simulink model "CSAD_PIDcontroller_ny"  (R2016b)
settings: Solver=ode3  StartTime=0.0  StopTime=tend  FixedStep=0.01  RelTol=1e-3  EnableMultiTasking=on
undefined symbols (not defined in the file): C, Cdn, Cdt, Cmn, d, D, depCur, des_pos, E, emfact, eps_c, epsilon, hd, hd2, Hoerner, I_s, k_cc, K_d_psi, K_d_x, K_d_y, K_i_psi, K_i_x, K_i_y, K_omega, K_p_psi, K_p_x, K_p_y, Kp, Kq, Kqr, Kt, Ktr, L, Max_Acceleration, Max_rotation, Max_thrust, moorLineProp, n_c, n_max, p_cc, P_max, Q_f0, Q_max, r0, r_cc, r_dot0, rBottomEnd, Rho, rhoCab, rhoWat, stiffSeafloor, T_psi, T_x, T_y, Thruster, Thruster_control, Thruster_lock, velCur, vessel, vesselABC ... (+7)
libraries: marine_gnc x9, dspmtrx3 x6, simulink x6, simulink_extras x3, marine_hydro x3
(part 1 of 5)
settings Model: Creator=JonBjoernoe  LastModifiedBy=silje
settings SolverCC: AlgebraicLoopSolver=LineSearch
settings OptimizationCC: LifeSpan=inf
settings DebuggingCC: SFUnexpectedBacktrackingDiag=warning  SFNoUnconditionalDefaultTransitionDiag=warning  SFExecutionAtInitializationDiag=none
settings ModelReferenceCC: ModelReferenceMinAlgLoopOccurrences=on
settings GRTTargetCC: TargetLangStandard=C89/C90 (ANSI)  GeneratePreprocessorConditionals=Disable all
settings ConfigComp: CovMetricSettings=dw  CovHtmlReporting=on  CovSaveCumulativeToWorkspaceVar=on  CovSaveSingleToWorkspaceVar=on  CovExternalEMLEnable=off

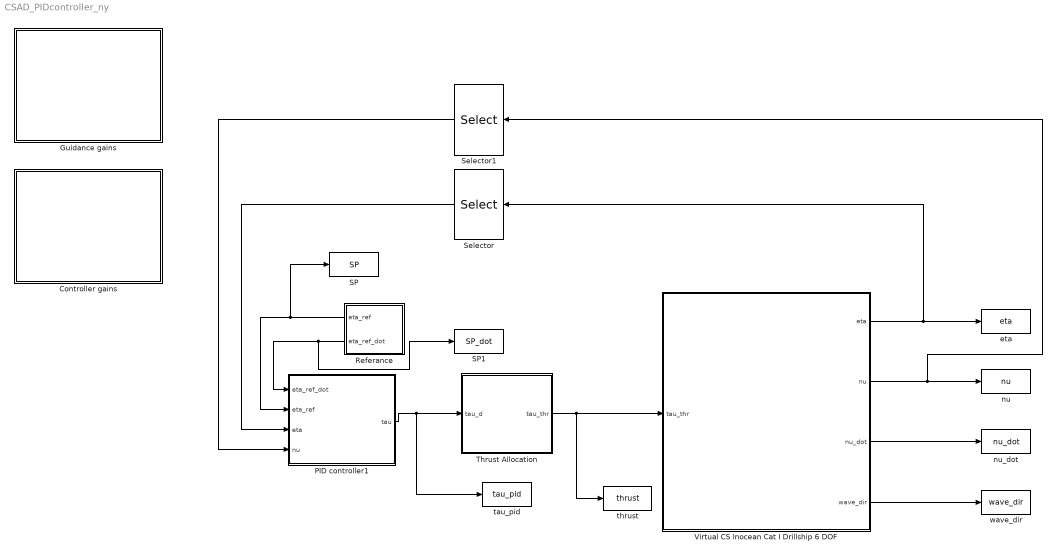
== system CSAD_PIDcontroller_ny ==
  Controller gains : Subsystem
  Guidance gains : Subsystem
  PID controller1 : Subsystem
  Referance : Subsystem
  SP : ToWorkspace  VariableName=SP  SaveFormat=Timeseries  SampleTime=-1
  SP1 : ToWorkspace  VariableName=SP_dot  SaveFormat=Timeseries  SampleTime=-1
  Selector : Selector  InputPortWidth=6  IndexOptions=Index vector (dialog)  Indices=[1 2 6]  OutputSizes=1
  Selector1 : Selector  InputPortWidth=6  IndexOptions=Index vector (dialog)  Indices=[1 2 6]  OutputSizes=1
  "Thrust Allocation  " : Subsystem
  Virtual CS Inocean Cat I Drillship 6 DOF : Subsystem  mask(CSAD with Turret-based thruster-assisted position mooring){eta_0=[0 0 0 0 0 0], nu_0=[0 0 0 0 0 0], wave_1_on_off=off, wave_2_on_off=on, Hs=1.5/90, beta_w=3.4907, omega_0=0.768*sqrt(90), current_on_off=on, nu_c=0.2/sqrt(90), beta_c=200, anchor_0=moorLineProp.bottomEnds, mooringLinesMeasurement_on_off=off, mooringLines_on_off=off}
      mask prompts: eta_0 "Initial eta"; nu_0 "Initial nu"; wave_1_on_off "Wave force (1st Order)"; wave_2_on_off "Wave drift force (2nd Order)"; Hs "Significant wave height [m] (Hs)"; beta_w "Mean wave direction [rad] (beta_w)"; omega_0 "Peak frequency [rad/s] (omega_0)"; current_on_off "Current"; nu_c "Current velocity [m/s] (nu_c)"; beta_c "Current direction [deg] (beta_c)"; anchor_0 "The anchor position matrix"; mooringLinesMeasurement_on_off "Mooring Lines' Measurement"; mooringLines_on_off "Mooring Lines"
      mask help:
      | This block implements the CS Inocean Cat I Drillship with 4 mooring lines. This is a simplified model. All the mooring lines are assumed to connect with the turret at the center of the turret (COT). The COT locates at the center of the ship.  Therefore, there are no moments from mooring lines.
      |
      | where
      | input 1:     <tau_thr> Thruster forces.
      | output 1:   <Wave direction> The direction of the waves.
      | output 2:   <eta> The position of the CSAD.
      | output 3:   <nu> The velocity of the CSAD.
      | output 4:   <T_moor> The tension vector in every mooring line.
      |
      | Copyright (C) 2016, NTNU, Trondheim, Norway
      | Author: Jon Bjørnø (CSAD) and Zhengru Ren (mooring)
  eta : ToWorkspace  VariableName=eta  SaveFormat=Timeseries  SampleTime=-1
  nu : ToWorkspace  VariableName=nu  SaveFormat=Timeseries  SampleTime=-1
  nu_dot : ToWorkspace  VariableName=nu_dot  SaveFormat=Timeseries  SampleTime=-1
  tau_pid : ToWorkspace  VariableName=tau_pid  SaveFormat=Timeseries  SampleTime=-1
  thrust : ToWorkspace  VariableName=thrust  SaveFormat=Timeseries  SampleTime=-1
  wave_dir : ToWorkspace  VariableName=wave_dir  SaveFormat=Timeseries  SampleTime=-1
  wires:
  Virtual CS Inocean Cat I Drillship 6 DOF/1(eta) -> Selector/1, eta/1
  Virtual CS Inocean Cat I Drillship 6 DOF/2(nu) -> nu/1, Selector1/1
  Virtual CS Inocean Cat I Drillship 6 DOF/3(nu_dot) -> nu_dot/1
  Virtual CS Inocean Cat I Drillship 6 DOF/4(wave_dir) -> wave_dir/1
  "Thrust Allocation  "/1(tau_thr) -> thrust/1, Virtual CS Inocean Cat I Drillship 6 DOF/1(tau_thr)
  PID controller1/1(tau) -> tau_pid/1, "Thrust Allocation  "/1(tau_d)
  Selector/1 -> PID controller1/3(eta)
  Selector1/1 -> PID controller1/4(nu)
  Referance/1(eta_ref) -> SP/1, PID controller1/2(eta_ref)
  Referance/2(eta_ref_dot) -> SP1/1, PID controller1/1(eta_ref_dot)

== system CSAD_PIDcontroller_ny/Controller gains ==
  Constant : Constant  Value=K_p_x
  Constant1 : Constant  Value=K_p_y
  Constant2 : Constant  Value=K_p_psi
  Constant3 : Constant  Value=K_i_x
  Constant4 : Constant  Value=K_i_y
  Constant5 : Constant  Value=K_i_psi
  Constant6 : Constant  Value=K_d_x
  Constant7 : Constant  Value=K_d_y
  Constant8 : Constant  Value=K_d_psi
  Create Diagonal Matrix : dspmtrx3/Create Diagonal Matrix
  Create Diagonal Matrix1 : dspmtrx3/Create Diagonal Matrix
  Create Diagonal Matrix2 : dspmtrx3/Create Diagonal Matrix
  Mux : Mux  Inputs=3
  Mux1 : Mux  Inputs=3
  Mux2 : Mux  Inputs=3
  tag scope: K_d=global, K_i=global, K_p=global
  wires:
  Mux/1 -> Create Diagonal Matrix/1
  Constant/1 -> Mux/1
  Constant1/1 -> Mux/2
  Constant2/1 -> Mux/3
  Mux1/1 -> Create Diagonal Matrix1/1
  Create Diagonal Matrix/1 -> [K_p]
  Create Diagonal Matrix1/1 -> [K_i]
  Mux2/1 -> Create Diagonal Matrix2/1
  Create Diagonal Matrix2/1 -> [K_d]
  Constant3/1 -> Mux1/1
  Constant4/1 -> Mux1/2
  Constant5/1 -> Mux1/3
  Constant6/1 -> Mux2/1
  Constant7/1 -> Mux2/2
  Constant8/1 -> Mux2/3

== system CSAD_PIDcontroller_ny/Guidance gains ==
  Constant : Constant  Value=w_x
  Constant1 : Constant  Value=w_y
  Constant2 : Constant  Value=w_psi
  Constant3 : Constant  Value=zeta_x
  Constant4 : Constant  Value=zeta_y
  Constant5 : Constant  Value=zeta_psi
  Constant6 : Constant  Value=1/T_x
  Constant7 : Constant  Value=1/T_y
  Constant8 : Constant  Value=1/T_psi
  Create Diagonal Matrix : dspmtrx3/Create Diagonal Matrix
  Create Diagonal Matrix1 : dspmtrx3/Create Diagonal Matrix
  Create Diagonal Matrix2 : dspmtrx3/Create Diagonal Matrix
  Mux : Mux  Inputs=3
  Mux1 : Mux  Inputs=3
  Mux2 : Mux  Inputs=3
  tag scope: Af=global, omega=global, zeta=global
  wires:
  Mux/1 -> Create Diagonal Matrix/1
  Constant/1 -> Mux/1
  Constant1/1 -> Mux/2
  Constant2/1 -> Mux/3
  Mux1/1 -> Create Diagonal Matrix1/1
  Constant3/1 -> Mux1/1
  Constant4/1 -> Mux1/2
  Constant5/1 -> Mux1/3
  Create Diagonal Matrix/1 -> [omega]
  Create Diagonal Matrix1/1 -> [zeta]
  Mux2/1 -> Create Diagonal Matrix2/1
  Constant6/1 -> Mux2/1
  Constant7/1 -> Mux2/2
  Constant8/1 -> Mux2/3
  Create Diagonal Matrix2/1 -> [Af]

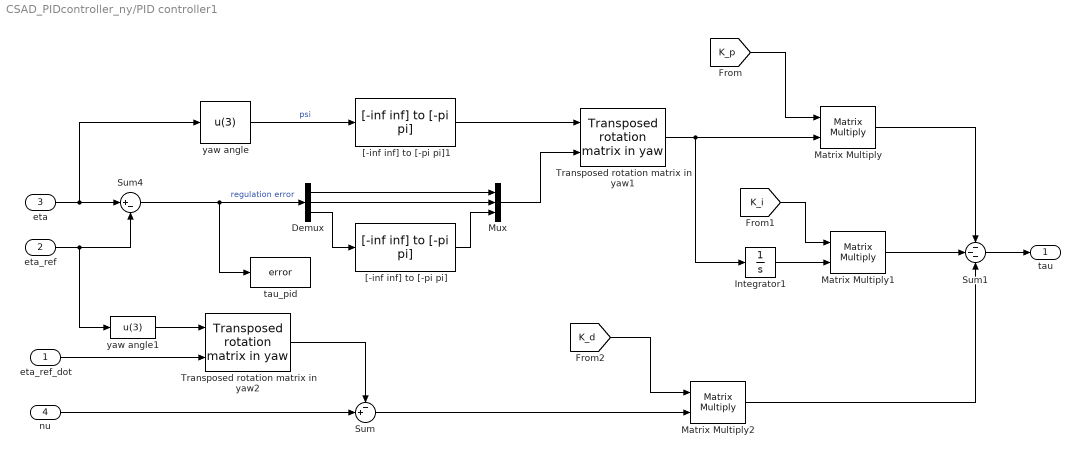
== system CSAD_PIDcontroller_ny/PID controller1 ==
  eta_ref_dot : Inport
  eta_ref : Inport  Port=2
  eta : Inport  Port=3
  nu : Inport  Port=4
  Demux : Demux  Outputs=3
  Integrator1 : Integrator
  Matrix Multiply : Product  Multiplication=Matrix(*)
  Matrix Multiply1 : Product  Multiplication=Matrix(*)
  Matrix Multiply2 : Product  Multiplication=Matrix(*)
  Mux : Mux  Inputs=3
  Sum : Sum  Inputs=-+|
  Sum1 : Sum  Inputs=---  SaturateOnIntegerOverflow=on  InputSameDT=on  OutDataTypeStr=Inherit: Same as first input
  Sum4 : Sum  Inputs=|+-  SaturateOnIntegerOverflow=on  InputSameDT=on  OutDataTypeStr=Inherit: Same as first input
  Transposed rotation matrix in yaw1 : marine_gnc/Models/ Kinematics/Transposed rotation  matrix in yaw
  Transposed rotation matrix in yaw2 : marine_gnc/Models/ Kinematics/Transposed rotation  matrix in yaw
  "[-inf inf] to [-pi pi]" : marine_gnc/Utilities/Math Operations/[-inf inf] to [-pi pi]
  "[-inf inf] to [-pi pi]1" : marine_gnc/Utilities/Math Operations/[-inf inf] to [-pi pi]
  tau_pid : ToWorkspace  VariableName=error  SaveFormat=Timeseries  SampleTime=-1
  yaw angle : Fcn  Expr=u(3)
  yaw angle1 : Fcn  Expr=u(3)
  tau : Outport  InitialOutput=0
  wires:
  Demux/2 -> Mux/2
  Demux/1 -> Mux/1
  Mux/1 -> Transposed rotation matrix in yaw1/2
  Sum4/1 -> tau_pid/1, Demux/1  "regulation error"
  "[-inf inf] to [-pi pi]"/1 -> Mux/3
  yaw angle/1 -> "[-inf inf] to [-pi pi]1"/1  "psi"
  "[-inf inf] to [-pi pi]1"/1 -> Transposed rotation matrix in yaw1/1
  Demux/3 -> "[-inf inf] to [-pi pi]"/1
  Transposed rotation matrix in yaw1/1 -> Matrix Multiply/2, Integrator1/1
  Sum1/1 -> tau/1
  eta_ref/1 -> yaw angle1/1, Sum4/2
  eta/1 -> yaw angle/1, Sum4/1
  [K_p] -> Matrix Multiply/1
  Matrix Multiply/1 -> Sum1/1
  Integrator1/1 -> Matrix Multiply1/2
  Matrix Multiply1/1 -> Sum1/2
  [K_i] -> Matrix Multiply1/1
  [K_d] -> Matrix Multiply2/1
  Matrix Multiply2/1 -> Sum1/3
  eta_ref_dot/1 -> Transposed rotation matrix in yaw2/2
  yaw angle1/1 -> Transposed rotation matrix in yaw2/1
  nu/1 -> Sum/2
  Sum/1 -> Matrix Multiply2/2
  Transposed rotation matrix in yaw2/1 -> Sum/1

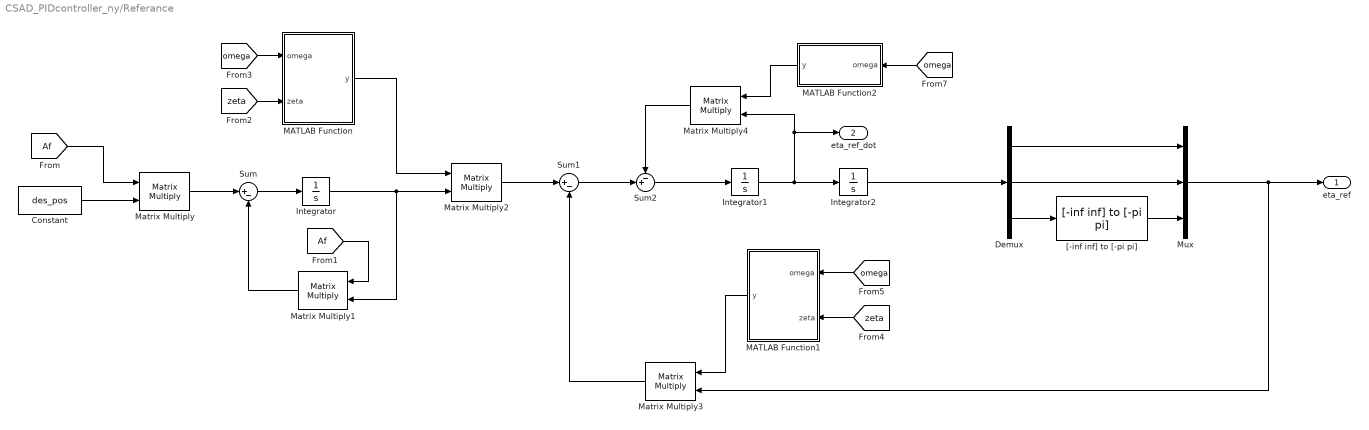
== system CSAD_PIDcontroller_ny/Referance ==
  Constant : Constant  Value=des_pos
  Demux : Demux  Outputs=3
  Integrator : Integrator
  Integrator1 : Integrator
  Integrator2 : Integrator
  MATLAB Function : MATLAB Function  TreatAsAtomicUnit=on
  MATLAB Function1 : MATLAB Function  TreatAsAtomicUnit=on
  MATLAB Function2 : MATLAB Function  TreatAsAtomicUnit=on
  Matrix Multiply{,1..4} (5 alike) : Product  Multiplication=Matrix(*)
  Mux : Mux  Inputs=3
  Sum : Sum  Inputs=|+-
  Sum1 : Sum  Inputs=|+-
  Sum2 : Sum  Inputs=-+|
  "[-inf inf] to [-pi pi]" : marine_gnc/Utilities/Math Operations/[-inf inf] to [-pi pi]
  eta_ref : Outport
  eta_ref_dot : Outport  Port=2
  wires:
  Constant/1 -> Matrix Multiply/2
  [Af] -> Matrix Multiply/1
  Matrix Multiply/1 -> Sum/1
  Sum/1 -> Integrator/1
  Matrix Multiply1/1 -> Sum/2
  [Af] -> Matrix Multiply1/1
  Integrator/1 -> Matrix Multiply2/2, Matrix Multiply1/2
  [zeta] -> MATLAB Function/2(zeta)
  [omega] -> MATLAB Function/1(omega)
  MATLAB Function/1(y) -> Matrix Multiply2/1
  Matrix Multiply2/1 -> Sum1/1
  Sum1/1 -> Sum2/2
  Sum2/1 -> Integrator1/1
  Integrator1/1 -> eta_ref_dot/1, Matrix Multiply4/2, Integrator2/1
  [zeta] -> MATLAB Function1/2(zeta)
  [omega] -> MATLAB Function1/1(omega)
  MATLAB Function1/1(y) -> Matrix Multiply3/1
  Matrix Multiply3/1 -> Sum1/2
  [omega] -> MATLAB Function2/1(omega)
  MATLAB Function2/1(y) -> Matrix Multiply4/1
  Matrix Multiply4/1 -> Sum2/1
  Demux/3 -> "[-inf inf] to [-pi pi]"/1
  "[-inf inf] to [-pi pi]"/1 -> Mux/3
  Demux/2 -> Mux/2
  Demux/1 -> Mux/1
  Integrator2/1 -> Demux/1
  Mux/1 -> Matrix Multiply3/2, eta_ref/1

== system CSAD_PIDcontroller_ny/Thrust Allocation   ==
  tau_d : Inport
  "Parameters From initfile distributed " : Subsystem
  T(F,alpha) : Subsystem
  Thrust allocation1 : Subsystem
  "Thruster control " : Subsystem
  tau_thr : Outport
  wires:
  T(F,alpha)/1(Commanded tau) -> tau_thr/1
  tau_d/1 -> Thrust allocation1/1(tau)
  "Thruster control "/2(Commanded angle) -> T(F,alpha)/2(Commanded angle), Thrust allocation1/2(Angles)
  Thrust allocation1/1(Td & angle) -> "Thruster control "/1("Desired thrust and angle ")
  "Thruster control "/1("Commanded thrust ") -> T(F,alpha)/1(Commanded thrust)

== system CSAD_PIDcontroller_ny/Virtual CS Inocean Cat I Drillship 6 DOF ==
  tau_thr : Inport
  3 to 6 DOF : marine_gnc/Models/ Kinetics /Support/3 to 6 DOF  SystemSampleTime=-1
  6 DOF DP model (zero speed model with fluid memory) : Subsystem  mask(6 DOF zero speed model){ABC=vesselABC, rho=1025, Axc=0.9*vessel.main.T*vessel.main.B, Ayc=0.9*vessel.main.T*vessel.main.Lpp, CX=1, CY_2D=Hoerner(vessel.main.B,vessel.main.T), Bv=vessel.Bv(:,:,1)}
      mask prompts: ABC "Structure containing model parameters and the fluid memory effects"; rho "Density of water (kg/m3)"; Axc "Frontal projected current area Axc (m2)"; Ayc "Laterall projected current area Ayc (m2)"; CX "Current (drag) coefficient in surge CX"; CY_2D "2D drag coefficient in sway CY_2D"; Bv "Linear viscous damping matrix"
      mask help: System block containing the zero speed 6 DOF equations of motion including fluid memory effetcs.
  Current : Subsystem
  Current direction (deg) : Constant  Value=beta_c
  Current speed (m/s) : Constant  Value=nu_c
  FEM mooring : Subsystem  mask(Mooring Force Model){r_0=moorLineProp.bottomEnds}
      mask prompts: r_0 "The anchor position matrix"
      mask help:
      | This block implements the mooring forces with catenary equations. There are 8 mooring lines in this mooring system. This is a simplified model. All the mooring lines are assumed to connect with the turret at the center of the turret (COT). The COT locates at the center of the ship.  Therefore, there are no moments from mooring lines.
      |
      | where
      | input 1:    <eta> The position of the turrent terminal point.
      | output 1:   <tau_moor> The total mooring forces in 6DOF. The moments in roll, pitch, and yaw are zeros.
      | output 2:   <T_moor> The tension vector in every mooring lines.
      |
      | Copyright (C) 2015, NTNU, Trondheim, Norway
      | Author: Zhengru Ren
      | Edited: Jon Bjørnø 2016
      mask DialogControl Container2 Prompt: Parameters
  Waves : Subsystem
  current : ToWorkspace  VariableName=current  SaveFormat=Timeseries  SampleTime=-1
  "currentForce on/off " : Gain  Gain=current_on_off
  mooringLines on/off : Gain  Gain=mooringLines_on_off
  wave : ToWorkspace  VariableName=wave  SaveFormat=Timeseries  SampleTime=-1
  eta : Outport
  nu : Outport  Port=2
  nu_dot : Outport  Port=3
  wave_dir : Outport  Port=4
  wires:
  6 DOF DP model (zero speed model with fluid memory)/2(nu) -> nu/1
  tau_thr/1 -> 3 to 6 DOF/1
  3 to 6 DOF/1 -> 6 DOF DP model (zero speed model with fluid memory)/2(tau_thr)
  FEM mooring/1(tau_moor) -> mooringLines on/off/1
  "currentForce on/off "/1 -> current/1, 6 DOF DP model (zero speed model with fluid memory)/3(nu_c)
  Current/1(nu_c) -> "currentForce on/off "/1
  Current speed (m/s)/1 -> Current/2(V_c (m/s))
  Current direction (deg)/1 -> Current/1(beta_c (deg))
  6 DOF DP model (zero speed model with fluid memory)/3(nu_dot) -> nu_dot/1
  6 DOF DP model (zero speed model with fluid memory)/1(eta) -> Waves/1(eta), FEM mooring/1(eta), eta/1
  Waves/1(wave_dir) -> wave_dir/1
  Waves/2(tau_wave) -> wave/1, 6 DOF DP model (zero speed model with fluid memory)/1(tau_wave)
  mooringLines on/off/1 -> 6 DOF DP model (zero speed model with fluid memory)/4(tau_mooring)

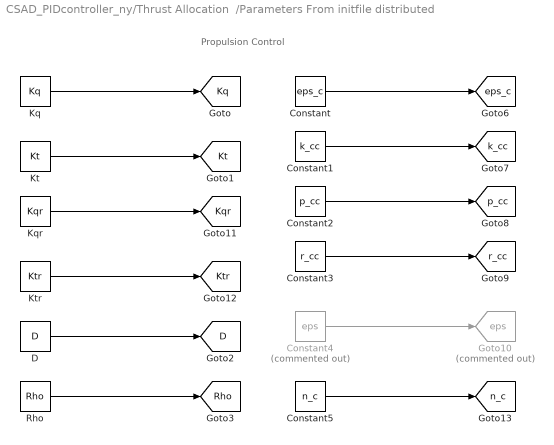
== system CSAD_PIDcontroller_ny/Thrust Allocation  /Parameters From initfile distributed  ==
  note: Propulsion Control
  Constant : Constant  Value=eps_c
  Constant1 : Constant  Value=k_cc
  Constant2 : Constant  Value=p_cc
  Constant3 : Constant  Value=r_cc
  Constant4 : Constant  Commented=on  Value=eps
  Constant5 : Constant  Value=n_c
  D : Constant  Value=D
  Goto10 : Goto  Commented=on  GotoTag=eps  TagVisibility=global
  Kq : Constant  Value=Kq
  Kqr : Constant  Value=Kqr
  Kt : Constant  Value=Kt
  Ktr : Constant  Value=Ktr
  Rho : Constant  Value=Rho
  tag scope: D=global, Kq=global, Kqr=global, Kt=global, Ktr=global, Rho=global, eps_c=global, k_cc=global, n_c=global, p_cc=global, r_cc=global
  wires:
  Kq/1 -> [Kq]
  Kt/1 -> [Kt]
  D/1 -> [D]
  Rho/1 -> [Rho]
  Constant/1 -> [eps_c]
  Constant1/1 -> [k_cc]
  Constant2/1 -> [p_cc]
  Constant3/1 -> [r_cc]
  Constant4/1 -> Goto10/1
  Kqr/1 -> [Kqr]
  Ktr/1 -> [Ktr]
  Constant5/1 -> [n_c]

== system CSAD_PIDcontroller_ny/Thrust Allocation  /T(F,alpha) ==
  Commanded thrust : Inport
  Commanded angle : Inport  Port=2
  MATLAB Function : MATLAB Function  TreatAsAtomicUnit=on
  Radians to Degrees : simulink_extras/Transformations/Radians to Degrees
  X-position Thruster : Constant  Value=[Thruster.T1(1) Thruster.T2(1) Thruster.T3(1) Thruster.T4(1) Thruster.T5(1) Thruster.T6(1)]
  Y-position Thruster : Constant  Value=[Thruster.T1(2) Thruster.T2(2) Thruster.T3(2) Thruster.T4(2) Thruster.T5(2) Thruster.T6(2)]
  Commanded tau : Outport
  wires:
  Commanded angle/1 -> Radians to Degrees/1
  X-position Thruster/1 -> MATLAB Function/3(PosX)
  Y-position Thruster/1 -> MATLAB Function/4(PosY)
  MATLAB Function/1(actual_tau) -> Commanded tau/1
  Commanded thrust/1 -> MATLAB Function/1(thrust_actual)
  Radians to Degrees/1 -> MATLAB Function/2(alpha_actual)

== system CSAD_PIDcontroller_ny/Thrust Allocation  /Thrust allocation1 ==
  tau : Inport
  Angles : Inport  Port=2
  "  Thrust calculated" : Selector  InputPortWidth=12  IndexOptions=Index vector (dialog)  Indices=[7 8 9 10 11 12]  OutputSizes=1
  " Angle calculated" : Selector  InputPortWidth=12  IndexOptions=Index vector (dialog)  Indices=[1 2 3 4 5 6]  OutputSizes=1
  Choosing Fixed / Azimuth angle : Switch  Threshold=1
  Constant to avoid singularities : Constant  Value=eps
  For Each Subsystem : Subsystem  TreatAsAtomicUnit=on
  Mux : Mux  Inputs=3
  Mux2 : Mux  Inputs=2
  Radians to Degrees : simulink_extras/Transformations/Radians to Degrees
  Switch Azimuth/Fixed angles : Constant  Value=Thruster_lock
  Thrust and angle specified : Selector  InputPortWidth=12  IndexOptions=Index vector (dialog)  Indices=[7 1 8 2 9 3 10 4 11 5 12 6]  OutputSizes=1
  ThrustAllocation_Pseudoinverse : S-Function  FunctionName=thrustallocationPseudo  Parameters=Thruster,C  SFunctionDeploymentMode=off  EnableBusSupport=off
      settings: AttributesFormatString=%<Commented>
  constant angle : Constant  Value=[Thruster.T1(3) Thruster.T2(3) Thruster.T3(3) Thruster.T4(3) Thruster.T5(3) Thruster.T6(3)]
  Td & angle : Outport
  wires:
  Switch Azimuth/Fixed angles/1 -> Choosing Fixed / Azimuth angle/2
  Constant to avoid singularities/1 -> Mux/3
  " Angle calculated"/1 -> Choosing Fixed / Azimuth angle/1
  Thrust and angle specified/1 -> Td & angle/1
  Mux2/1 -> Thrust and angle specified/1
  tau/1 -> Mux/1
  Choosing Fixed / Azimuth angle/1 -> For Each Subsystem/1(Desired Angle)
  Angles/1 -> Radians to Degrees/1
  For Each Subsystem/1("angle ") -> Mux2/1
  constant angle/1 -> For Each Subsystem/2("initial angle "), Choosing Fixed / Azimuth angle/3
  Radians to Degrees/1 -> Mux/2
  ThrustAllocation_Pseudoinverse/1 -> " Angle calculated"/1, "  Thrust calculated"/1
  Mux/1 -> ThrustAllocation_Pseudoinverse/1
  "  Thrust calculated"/1 -> Mux2/2

== system CSAD_PIDcontroller_ny/Thrust Allocation  /Thruster control  ==
  "Desired thrust and angle " : Inport
  Demux : Demux  Outputs=12
  Mux : Mux  Inputs=12
  Selecting Actual thrust : Selector  InputPortWidth=12  IndexOptions=Index vector (dialog)  Indices=[1 3 5 7 9 11]  OutputSizes=1
  Selecting actual angle : Selector  InputPortWidth=12  IndexOptions=Index vector (dialog)  Indices=[2 4 6 8 10 12]  OutputSizes=1
  Subsystem : Subsystem
  Subsystem1 : Subsystem  Commented=through
  Thruster 1 : Subsystem
      settings: AttributesFormatString=%<MinAlgLoopOccurrences>
  Thruster 2 : Subsystem
      settings: AttributesFormatString=%<MinAlgLoopOccurrences>
  Thruster 3 : Subsystem
      settings: AttributesFormatString=%<MinAlgLoopOccurrences>
  Thruster 4 : Subsystem
      settings: AttributesFormatString=%<MinAlgLoopOccurrences>
  Thruster 5 : Subsystem
      settings: AttributesFormatString=%<MinAlgLoopOccurrences>
  Thruster 6 : Subsystem
      settings: AttributesFormatString=%<MinAlgLoopOccurrences>
  "Commanded thrust " : Outport
  Commanded angle : Outport  Port=2
  wires:
  "Desired thrust and angle "/1 -> Demux/1
  Demux/3 -> Thruster 2/1(Desired thrust 1)
  Demux/4 -> Thruster 2/2(Desired Angle)
  Demux/5 -> Thruster 3/1(Desired thrust 1)
  Demux/6 -> Thruster 3/2(Desired Angle)
  Demux/7 -> Thruster 4/1(Desired thrust 1)
  Demux/8 -> Thruster 4/2(Desired Angle)
  Demux/9 -> Thruster 5/1(Desired thrust 1)
  Demux/10 -> Thruster 5/2(Desired Angle)
  Demux/11 -> Thruster 6/1(Desired thrust 1)
  Demux/12 -> Thruster 6/2(Desired Angle)
  Thruster 1/1(Commanded thrust 1) -> Mux/1
  Thruster 2/1(Commanded thrust 1) -> Mux/3
  Thruster 2/2(Commanded angle) -> Mux/4
  Thruster 3/1("Commanded thrust ") -> Mux/5
  Thruster 3/2(Commanded angle) -> Mux/6
  Thruster 4/1("Commanded thrust ") -> Mux/7
  Thruster 4/2(Commanded angle) -> Mux/8
  Thruster 5/1(Commanded thrust 1) -> Mux/9
  Thruster 5/2(Commanded angle) -> Mux/10
  Thruster 6/1(Commanded thrust 1) -> Mux/11
  Thruster 6/2(Commanded angle) -> Mux/12
  Selecting actual angle/1 -> Subsystem1/1(Calculated angles)
  Mux/1 -> Selecting Actual thrust/1, Selecting actual angle/1
  Demux/2 -> Thruster 1/2(Desired Angle)
  Thruster 1/2(Commanded angle) -> Mux/2
  Subsystem1/1(Commanded angles) -> Commanded angle/1
  Subsystem/1(Thrust from model) -> "Commanded thrust "/1
  Selecting Actual thrust/1 -> Subsystem/1(Calculated thrust)
  Demux/1 -> Thruster 1/1(Desired thrust 1)

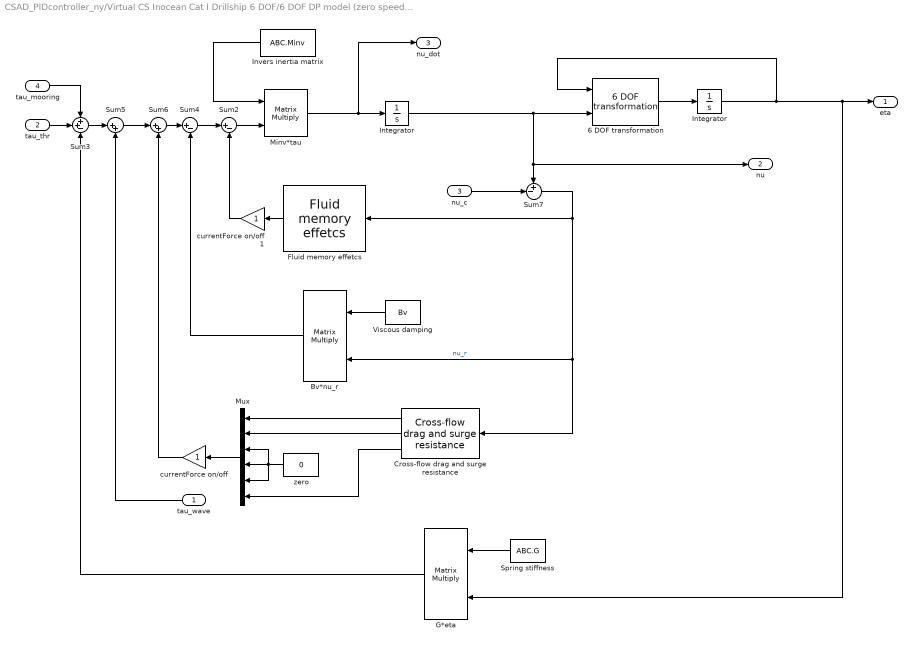
== system CSAD_PIDcontroller_ny/Virtual CS Inocean Cat I Drillship 6 DOF/6 DOF DP model (zero speed model with fluid memory) ==
  tau_wave : Inport
  tau_thr : Inport  Port=2
  nu_c : Inport  Port=3
  tau_mooring : Inport  Port=4
  6 DOF transformation : marine_gnc/Models/ Kinematics/6 DOF transformation
  Bv*nu_r : Product  Multiplication=Matrix(*)  SaturateOnIntegerOverflow=on  OutDataTypeStr=Inherit: Same as first input
  Cross-flow drag and surge resistance : marine_hydro/Hydro Library/Cross-flow drag and surge resistance  N=20  Lpp=vessel.main.Lpp  CD=CY_2D  Cx=CX  Ax=Axc  Ay=Ayc  rho_w=rho
  Fluid memory effetcs : marine_hydro/Hydro Library/6 DOF DP model  (zero speed model with fluid memory)/Fluid memory effetcs
  G*eta : Product  Multiplication=Matrix(*)  SaturateOnIntegerOverflow=on  OutDataTypeStr=Inherit: Same as first input
  Integrator : Integrator  InitialCondition=eta_0
  "Integrator " : Integrator  InitialCondition=nu_0
  Invers inertia matrix : Constant  Value=ABC.Minv
  Minv*tau : Product  Inputs=**  Multiplication=Matrix(*)  SaturateOnIntegerOverflow=on  OutDataTypeStr=Inherit: Same as first input
  Mux : Mux  Inputs=6
  Spring stiffness : Constant  Value=ABC.G
  Sum2 : Sum  Inputs=|+-  SaturateOnIntegerOverflow=on
  Sum3 : Sum  Inputs=++-  SaturateOnIntegerOverflow=on
  Sum4 : Sum  Inputs=|+-  SaturateOnIntegerOverflow=on
  Sum5 : Sum  Inputs=|++  SaturateOnIntegerOverflow=on
  Sum6 : Sum  Inputs=|++  SaturateOnIntegerOverflow=on
  Sum7 : Sum  Inputs=+-|  SaturateOnIntegerOverflow=on
  Viscous damping : Constant  Value=Bv
  "currentForce on/off " : Gain
  currentForce on/off 1 : Gain
  zero : Constant  Value=0
  eta : Outport
  nu : Outport  Port=2
  nu_dot : Outport  Port=3
  wires:
  6 DOF transformation/1 -> Integrator/1
  Cross-flow drag and surge resistance/1 -> Mux/1
  tau_wave/1 -> Sum5/2
  Sum5/1 -> Sum6/1
  Integrator/1 -> 6 DOF transformation/1, eta/1, G*eta/2
  Spring stiffness/1 -> G*eta/1
  Sum6/1 -> Sum4/1
  "Integrator "/1 -> 6 DOF transformation/2, nu/1, Sum7/1
  Sum7/1 -> Fluid memory effetcs/1, Cross-flow drag and surge resistance/1, Bv*nu_r/2  "nu_r"
  Mux/1 -> "currentForce on/off "/1
  Viscous damping/1 -> Bv*nu_r/1
  Sum4/1 -> Sum2/1
  Cross-flow drag and surge resistance/3 -> Mux/6
  zero/1 -> Mux/4, Mux/3, Mux/5
  Sum2/1 -> Minv*tau/2
  Sum3/1 -> Sum5/1
  Fluid memory effetcs/1 -> currentForce on/off 1/1
  Invers inertia matrix/1 -> Minv*tau/1
  nu_c/1 -> Sum7/2
  Bv*nu_r/1 -> Sum4/2
  Cross-flow drag and surge resistance/2 -> Mux/2
  Minv*tau/1 -> nu_dot/1, "Integrator "/1
  tau_thr/1 -> Sum3/2
  tau_mooring/1 -> Sum3/1
  "currentForce on/off "/1 -> Sum6/2
  currentForce on/off 1/1 -> Sum2/2
  G*eta/1 -> Sum3/3

== system CSAD_PIDcontroller_ny/Virtual CS Inocean Cat I Drillship 6 DOF/Current ==
  beta_c (deg) : Inport
  V_c (m/s) : Inport  Port=2
  Gain : Gain  Gain=pi/180
  Mux : Mux  Inputs=6
  Product : Product  RndMeth=Zero
  Product1 : Product  RndMeth=Zero
  cos : Trigonometry  Operator=cos
  deg to 180/180 : marine_gnc/Utilities/Math Operations/deg to 180//180
  sin : Trigonometry
  zero : Constant  Value=0
  nu_c : Outport
  wires:
  sin/1 -> Product1/1
  cos/1 -> Product/1
  Product1/1 -> Mux/2
  zero/1 -> Mux/6, Mux/5, Mux/4, Mux/3
  V_c (m/s)/1 -> Product/2, Product1/2
  Gain/1 -> cos/1, sin/1
  Product/1 -> Mux/1
  Mux/1 -> nu_c/1
  beta_c (deg)/1 -> deg to 180/180/1
  deg to 180/180/1 -> Gain/1

== system CSAD_PIDcontroller_ny/Virtual CS Inocean Cat I Drillship 6 DOF/FEM mooring ==
  eta : Inport
  3 DOF transformation : MATLAB Function  TreatAsAtomicUnit=on
  Gain{,1..3} (4 alike) : Gain  Gain=0
  Mooring Line 1 : Subsystem
  Mooring Line 2 : Subsystem
  Mooring Line 3 : Subsystem
  Mooring Line 4 : Subsystem
  Mooring Line 5 : Subsystem
  Mooring Line 6 : Subsystem
  Mooring Line 7 : Subsystem
  Mooring Line 8 : Subsystem
  Selector : Selector  InputPortWidth=6  IndexOptions=Index vector (dialog)  Indices=[1 2 3]  OutputSizes=1
  Sum1 : Sum  Inputs=++++++++  SaturateOnIntegerOverflow=on  InputSameDT=on  OutDataTypeStr=Inherit: Same as first input
  eta1 : InportShadow
  mooring : ToWorkspace  VariableName=mooring  SaveFormat=Timeseries  SampleTime=-1
  scaling_eta : MATLAB Function  TreatAsAtomicUnit=on
  scaling_eta1 : MATLAB Function  TreatAsAtomicUnit=on
  scaling_tau : MATLAB Function  TreatAsAtomicUnit=on
  tau_moor : Outport
  wires:
  Sum1/1 -> 3 DOF transformation/2(tau_n)
  eta/1 -> scaling_eta1/1(u)
  eta1/1 -> Selector/1
  scaling_eta1/1(y) -> 3 DOF transformation/1(eta)
  scaling_tau/1(y) -> tau_moor/1
  Mooring Line 1/1("tau_moor [H_x, H_y, V]") -> mooring/1, Sum1/1
  Mooring Line 5/1("tau_moor [H_x, H_y, V]") -> Gain3/1
  Mooring Line 6/1("tau_moor [H_x, H_y, V]") -> Gain2/1
  Mooring Line 7/1("tau_moor [H_x, H_y, V]") -> Gain1/1
  Mooring Line 8/1("tau_moor [H_x, H_y, V]") -> Gain/1
  scaling_eta/1(y) -> Mooring Line 8/1(eta), Mooring Line 7/1(eta), Mooring Line 6/1(eta), Mooring Line 5/1(eta), Mooring Line 4/1(eta), Mooring Line 3/1(eta), Mooring Line 2/1(eta), Mooring Line 1/1(eta)
  Selector/1 -> scaling_eta/1(u)
  3 DOF transformation/1(tau_b) -> scaling_tau/1(u)
  Gain/1 -> Sum1/8
  Gain1/1 -> Sum1/7
  Gain2/1 -> Sum1/6
  Gain3/1 -> Sum1/5
  Mooring Line 4/1("tau_moor [H_x, H_y, V]") -> Sum1/4
  Mooring Line 3/1("tau_moor [H_x, H_y, V]") -> Sum1/3
  Mooring Line 2/1("tau_moor [H_x, H_y, V]") -> Sum1/2

== system CSAD_PIDcontroller_ny/Virtual CS Inocean Cat I Drillship 6 DOF/Waves ==
  eta : Inport
  Sum : Sum  Inputs=++|
  Wave loads (U=0) : marine_hydro/Hydro Library/Wave loads (U=0)
  Waves : marine_gnc/Environment/Waves/Waves  spectrum_type=Jonswap  disp_flag=off  plot_spectrum=off  plot_realization=off  hs=Hs  omega_peak=omega_0  psi_mean=beta_w  gamma=0  spread=2  depth=1000  nfreq=20  ndir=1  energylim=0.005  freq_cutoff=3  dir_cutoff=0  rand_seed=0  rand_freq=on  rand_dir=on  Zeta_a=0  Omega=0  Phase=0  Wavenum=0  Psi=0
  waveDriftForce on/off : Gain  Gain=wave_2_on_off
  waveForce on/off : Gain  Gain=wave_1_on_off
  wave_dir : Outport
  tau_wave : Outport  Port=2
  wires:
  Waves/1 -> Wave loads (U=0)/2
  Wave loads (U=0)/1 -> waveForce on/off/1
  waveDriftForce on/off/1 -> Sum/1
  Wave loads (U=0)/2 -> waveDriftForce on/off/1
  waveForce on/off/1 -> Sum/2
  Waves/2 -> wave_dir/1
  eta/1 -> Wave loads (U=0)/1
  Sum/1 -> tau_wave/1

== system CSAD_PIDcontroller_ny/Thrust Allocation  /Thrust allocation1/For Each Subsystem ==
  Desired Angle : Inport  Partition=on  PartitionDimension=1  PartitionWidth=1
  "initial angle " : Inport  Port=2  Partition=on  PartitionDimension=1  PartitionWidth=1
  Degrees to Radians : simulink_extras/Transformations/Degrees to Radians
  Ensures fastest way is chosen : MATLAB Function  TreatAsAtomicUnit=on
  For Each : ForEach  DisableCoverage=on  IndexMode=One-based
  Integrator : Integrator  ExternalReset=either  InitialConditionSource=external
  MATLAB Function : MATLAB Function  TreatAsAtomicUnit=on
  Max Rotation Rate : Saturate  UpperLimit=Max_rotation  LowerLimit=-Max_rotation
  constant : Constant  Value=0
  "angle " : Outport  ConcatenationDimension=1
  wires:
  Degrees to Radians/1 -> MATLAB Function/1(angle)
  MATLAB Function/1(y) -> "angle "/1
  Integrator/1 -> Degrees to Radians/1, Ensures fastest way is chosen/2(actual)  "angle"
  "initial angle "/1 -> Integrator/3
  Max Rotation Rate/1 -> Integrator/1
  Ensures fastest way is chosen/1(psi_D) -> Max Rotation Rate/1
  Desired Angle/1 -> Ensures fastest way is chosen/1(desired)
  constant/1 -> Integrator/2

== system CSAD_PIDcontroller_ny/Thrust Allocation  /Thruster control /Subsystem ==
  Calculated thrust : Inport
  Demux : Demux  Outputs=6
  Mux : Mux  Inputs=6
  Saturation {1..6} (6 alike) : Saturate  UpperLimit=Max_thrust  LowerLimit=-Max_thrust
  Thrust from model : Outport
  wires:
  Calculated thrust/1 -> Demux/1
  Demux/1 -> Saturation 1/1
  Demux/2 -> Saturation 2/1
  Demux/3 -> Saturation 3/1
  Demux/4 -> Saturation 4/1
  Demux/5 -> Saturation 5/1
  Demux/6 -> Saturation 6/1
  Mux/1 -> Thrust from model/1
  Saturation 1/1 -> Mux/1
  Saturation 6/1 -> Mux/6
  Saturation 5/1 -> Mux/5
  Saturation 4/1 -> Mux/4
  Saturation 3/1 -> Mux/3
  Saturation 2/1 -> Mux/2

== system CSAD_PIDcontroller_ny/Thrust Allocation  /Thruster control /Subsystem1 ==
  Calculated angles : Inport
  Demux : Demux  Outputs=6
  Mux : Mux  Inputs=6
  Saturation {1..6} (6 alike) : Saturate  UpperLimit=pi  LowerLimit=-pi
  Commanded angles : Outport
  wires:
  Calculated angles/1 -> Demux/1
  Demux/1 -> Saturation 1/1
  Demux/2 -> Saturation 2/1
  Demux/3 -> Saturation 3/1
  Demux/4 -> Saturation 4/1
  Demux/5 -> Saturation 5/1
  Demux/6 -> Saturation 6/1
  Mux/1 -> Commanded angles/1
  Saturation 1/1 -> Mux/1
  Saturation 6/1 -> Mux/6
  Saturation 5/1 -> Mux/5
  Saturation 2/1 -> Mux/2
  Saturation 3/1 -> Mux/3
  Saturation 4/1 -> Mux/4

== system CSAD_PIDcontroller_ny/Thrust Allocation  /Thruster control /Thruster 1 ==
  Desired thrust 1 : Inport
  Desired Angle : Inport  Port=2
  Constant : Constant  Value=hd2.den{1,1}
  Constant1 : Constant  Value=hd2.num{1,1}
  Discrete Transfer Fcn : DiscreteTransferFcn  NumeratorSource=Input port  DenominatorSource=Input port  Denominator=[0.2 1]  SampleTime=0.01  a0EqualsOne=on
      settings: InputPortMap=u0,p1,p3
  Losses (placeholder) : Constant  Value=0
  Propeller Hydrodynamics : Subsystem
  Shaft dynamics : Subsystem
  Thruster control : Subsystem
  Commanded thrust 1 : Outport
  Commanded angle : Outport  Port=2
  wires:
  Losses (placeholder)/1 -> Propeller Hydrodynamics/1(env)
  Propeller Hydrodynamics/1(Ta) -> Commanded thrust 1/1
  Thruster control/1(Qc) -> Discrete Transfer Fcn/1
  Desired Angle/1 -> Commanded angle/1
  Constant1/1 -> Discrete Transfer Fcn/2
  Constant/1 -> Discrete Transfer Fcn/3
  Propeller Hydrodynamics/2(Qa) -> Shaft dynamics/2(Qa)
  Discrete Transfer Fcn/1 -> Shaft dynamics/1(Qm)
  Desired thrust 1/1 -> Thruster control/1("T_d ")
  Shaft dynamics/1(n) -> Thruster control/2(n), Propeller Hydrodynamics/2(n)

== system CSAD_PIDcontroller_ny/Thrust Allocation  /Thruster control /Thruster 2 ==
  Desired thrust 1 : Inport
  Desired Angle : Inport  Port=2
  Constant : Constant  Value=hd2.den{1,1}
  Constant1 : Constant  Value=hd2.num{1,1}
  Discrete Transfer Fcn : DiscreteTransferFcn  NumeratorSource=Input port  DenominatorSource=Input port  Denominator=[0.2 1]  SampleTime=0.01  a0EqualsOne=on
      settings: InputPortMap=u0,p1,p3
  Losses (placeholder) : Constant  Value=0
  Propeller Hydrodynamics : Subsystem
  Shaft dynamics : Subsystem
  Thruster control : Subsystem
  Commanded thrust 1 : Outport
  Commanded angle : Outport  Port=2
  wires:
  Losses (placeholder)/1 -> Propeller Hydrodynamics/1(env)
  Thruster control/1(Qc) -> Discrete Transfer Fcn/1
  Discrete Transfer Fcn/1 -> Shaft dynamics/1(Qm)
  Desired thrust 1/1 -> Thruster control/1("T_d ")
  Propeller Hydrodynamics/1(Ta) -> Commanded thrust 1/1
  Desired Angle/1 -> Commanded angle/1
  Constant1/1 -> Discrete Transfer Fcn/2
  Constant/1 -> Discrete Transfer Fcn/3
  Propeller Hydrodynamics/2(Qa) -> Shaft dynamics/2(Qa)
  Shaft dynamics/1(n) -> Thruster control/2(n), Propeller Hydrodynamics/2(n)

== system CSAD_PIDcontroller_ny/Thrust Allocation  /Thruster control /Thruster 3 ==
  Desired thrust 1 : Inport
  Desired Angle : Inport  Port=2
  Constant : Constant  Value=hd2.den{1,1}
  Constant1 : Constant  Value=hd2.num{1,1}
  Discrete Transfer Fcn : DiscreteTransferFcn  NumeratorSource=Input port  DenominatorSource=Input port  Denominator=[0.2 1]  SampleTime=0.01  a0EqualsOne=on
      settings: InputPortMap=u0,p1,p3
  Losses (placeholder) : Constant  Value=0
  Propeller Hydrodynamics : Subsystem
  Shaft dynamics : Subsystem
  Thruster control : Subsystem
  "Commanded thrust " : Outport
  Commanded angle : Outport  Port=2
  wires:
  Losses (placeholder)/1 -> Propeller Hydrodynamics/1(env)
  Thruster control/1(Qc) -> Discrete Transfer Fcn/1
  Discrete Transfer Fcn/1 -> Shaft dynamics/1(Qm)
  Desired thrust 1/1 -> Thruster control/1("T_d ")
  Propeller Hydrodynamics/1(Ta) -> "Commanded thrust "/1
  Desired Angle/1 -> Commanded angle/1
  Constant1/1 -> Discrete Transfer Fcn/2
  Constant/1 -> Discrete Transfer Fcn/3
  Propeller Hydrodynamics/2(Qa) -> Shaft dynamics/2(Qa)
  Shaft dynamics/1(n) -> Thruster control/2(n), Propeller Hydrodynamics/2(n)

== system CSAD_PIDcontroller_ny/Thrust Allocation  /Thruster control /Thruster 4 ==
  Desired thrust 1 : Inport
  Desired Angle : Inport  Port=2
  Constant : Constant  Value=hd2.den{1,1}
  Constant1 : Constant  Value=hd2.num{1,1}
  Discrete Transfer Fcn : DiscreteTransferFcn  NumeratorSource=Input port  DenominatorSource=Input port  Denominator=[0.2 1]  SampleTime=0.01  a0EqualsOne=on
      settings: InputPortMap=u0,p1,p3
  Losses (placeholder) : Constant  Value=0
  Propeller Hydrodynamics : Subsystem
  Shaft dynamics : Subsystem
  Thruster control : Subsystem
  "Commanded thrust " : Outport
  Commanded angle : Outport  Port=2
  wires:
  Losses (placeholder)/1 -> Propeller Hydrodynamics/1(env)
  Thruster control/1(Qc) -> Discrete Transfer Fcn/1
  Discrete Transfer Fcn/1 -> Shaft dynamics/1(Qm)
  Desired thrust 1/1 -> Thruster control/1("T_d ")
  Propeller Hydrodynamics/1(Ta) -> "Commanded thrust "/1
  Desired Angle/1 -> Commanded angle/1
  Constant1/1 -> Discrete Transfer Fcn/2
  Constant/1 -> Discrete Transfer Fcn/3
  Propeller Hydrodynamics/2(Qa) -> Shaft dynamics/2(Qa)
  Shaft dynamics/1(n) -> Thruster control/2(n), Propeller Hydrodynamics/2(n)

== system CSAD_PIDcontroller_ny/Thrust Allocation  /Thruster control /Thruster 5 ==
  Desired thrust 1 : Inport
  Desired Angle : Inport  Port=2
  Constant : Constant  Value=hd2.den{1,1}
  Constant1 : Constant  Value=hd2.num{1,1}
  Discrete Transfer Fcn : DiscreteTransferFcn  NumeratorSource=Input port  DenominatorSource=Input port  Denominator=[0.2 1]  SampleTime=0.01  a0EqualsOne=on
      settings: InputPortMap=u0,p1,p3
  Losses (placeholder) : Constant  Value=0
  Propeller Hydrodynamics : Subsystem
  Shaft dynamics : Subsystem
  Thruster control : Subsystem
  Commanded thrust 1 : Outport
  Commanded angle : Outport  Port=2
  wires:
  Losses (placeholder)/1 -> Propeller Hydrodynamics/1(env)
  Thruster control/1(Qc) -> Discrete Transfer Fcn/1
  Discrete Transfer Fcn/1 -> Shaft dynamics/1(Qm)
  Desired thrust 1/1 -> Thruster control/1("T_d ")
  Propeller Hydrodynamics/1(Ta) -> Commanded thrust 1/1
  Desired Angle/1 -> Commanded angle/1
  Constant1/1 -> Discrete Transfer Fcn/2
  Constant/1 -> Discrete Transfer Fcn/3
  Propeller Hydrodynamics/2(Qa) -> Shaft dynamics/2(Qa)
  Shaft dynamics/1(n) -> Thruster control/2(n), Propeller Hydrodynamics/2(n)

== system CSAD_PIDcontroller_ny/Thrust Allocation  /Thruster control /Thruster 6 ==
  Desired thrust 1 : Inport
  Desired Angle : Inport  Port=2
  Constant : Constant  Value=hd2.den{1,1}
  Constant1 : Constant  Value=hd2.num{1,1}
  Discrete Transfer Fcn : DiscreteTransferFcn  NumeratorSource=Input port  DenominatorSource=Input port  Denominator=[0.2 1]  SampleTime=0.01  a0EqualsOne=on
      settings: InputPortMap=u0,p1,p3
  Losses (placeholder) : Constant  Value=0
  Propeller Hydrodynamics : Subsystem
  Shaft dynamics : Subsystem
  Thruster control : Subsystem
  Commanded thrust 1 : Outport
  Commanded angle : Outport  Port=2
  wires:
  Losses (placeholder)/1 -> Propeller Hydrodynamics/1(env)
  Thruster control/1(Qc) -> Discrete Transfer Fcn/1
  Discrete Transfer Fcn/1 -> Shaft dynamics/1(Qm)
  Desired thrust 1/1 -> Thruster control/1("T_d ")
  Propeller Hydrodynamics/1(Ta) -> Commanded thrust 1/1
  Desired Angle/1 -> Commanded angle/1
  Constant1/1 -> Discrete Transfer Fcn/2
  Constant/1 -> Discrete Transfer Fcn/3
  Propeller Hydrodynamics/2(Qa) -> Shaft dynamics/2(Qa)
  Shaft dynamics/1(n) -> Thruster control/2(n), Propeller Hydrodynamics/2(n)

== system CSAD_PIDcontroller_ny/Virtual CS Inocean Cat I Drillship 6 DOF/FEM mooring/Mooring Line 1 ==
  eta : Inport
  Constant : Constant  Value=d
  Constant1 : Constant  Value=E
  Constant12 : Constant  Value=waterDepth(1)
  Constant14 : Constant  Value=emfact
  Constant15 : Constant  Value=rBottomEnd(:,1)
  Constant17 : Constant  Value=stiffSeafloor
  Constant2 : Constant  Value=L
  Constant3 : Constant  Value=velCur
  Constant4 : Constant  Value=rhoCab
  Constant5 : Constant  Value=rhoWat
  Constant6 : Constant  Value=Cmn
  Constant7 : Constant  Value=Cdt
  Constant8 : Constant  Value=Cdn
  Constant9 : Constant  Value=depCur
  FEM mooring cable : MATLAB Function  TreatAsAtomicUnit=on
  Scope : Scope
  To Workspace2 : ToWorkspace  VariableName=FtopPlot  SaveFormat=Timeseries  SampleTime=-1
  mo1 : ToWorkspace  VariableName=mooring_cabel1  SaveFormat=Timeseries  SampleTime=-1
  r0 : Integrator  InitialCondition=[r0(:,1);r_dot0(:,1)]
  "tau_moor [H_x, H_y, V]" : Outport
  wires:
  FEM mooring cable/1(state_dot) -> r0/1  "[r_dot;r_ddot]"
  Constant/1 -> FEM mooring cable/5(d)
  Constant1/1 -> FEM mooring cable/4(E)
  Constant2/1 -> FEM mooring cable/6(L)
  Constant4/1 -> FEM mooring cable/7(rhoCab)
  Constant5/1 -> FEM mooring cable/8(rhoWat)
  Constant6/1 -> FEM mooring cable/11(Cmn)
  Constant7/1 -> FEM mooring cable/12(Cdt)
  Constant8/1 -> FEM mooring cable/13(Cdn)
  Constant9/1 -> FEM mooring cable/14(depCur)
  Constant3/1 -> FEM mooring cable/15(velCur)
  r0/1 -> mo1/1, FEM mooring cable/1(state)  "[r;r_dot]"
  Constant14/1 -> FEM mooring cable/9(emfact)
  FEM mooring cable/2(Ftop) -> Scope/1, To Workspace2/1, "tau_moor [H_x, H_y, V]"/1
  Constant12/1 -> FEM mooring cable/16(waterDepth)
  Constant15/1 -> FEM mooring cable/2(rBottomEnd)
  Constant17/1 -> FEM mooring cable/10(stiffSeafloor)
  eta/1 -> FEM mooring cable/3(rTopEnd)

== system CSAD_PIDcontroller_ny/Virtual CS Inocean Cat I Drillship 6 DOF/FEM mooring/Mooring Line 2 ==
  eta : Inport
  Constant : Constant  Value=d
  Constant1 : Constant  Value=E
  Constant12 : Constant  Value=waterDepth(2)
  Constant14 : Constant  Value=emfact
  Constant15 : Constant  Value=rBottomEnd(:,2)
  Constant17 : Constant  Value=stiffSeafloor
  Constant2 : Constant  Value=L
  Constant3 : Constant  Value=velCur
  Constant4 : Constant  Value=rhoCab
  Constant5 : Constant  Value=rhoWat
  Constant6 : Constant  Value=Cmn
  Constant7 : Constant  Value=Cdt
  Constant8 : Constant  Value=Cdn
  Constant9 : Constant  Value=depCur
  FEM mooring cable : MATLAB Function  TreatAsAtomicUnit=on
  Scope : Scope
  To Workspace2 : ToWorkspace  VariableName=FtopPlot1  SaveFormat=Timeseries  SampleTime=-1
  mo2 : ToWorkspace  VariableName=mooring_cabel2  SaveFormat=Timeseries  SampleTime=-1
  r0 : Integrator  InitialCondition=[r0(:,2);r_dot0(:,2)]
  "tau_moor [H_x, H_y, V]" : Outport
  wires:
  FEM mooring cable/1(state_dot) -> r0/1  "[r_dot;r_ddot]"
  Constant/1 -> FEM mooring cable/5(d)
  Constant1/1 -> FEM mooring cable/4(E)
  Constant2/1 -> FEM mooring cable/6(L)
  Constant4/1 -> FEM mooring cable/7(rhoCab)
  Constant5/1 -> FEM mooring cable/8(rhoWat)
  Constant6/1 -> FEM mooring cable/11(Cmn)
  Constant7/1 -> FEM mooring cable/12(Cdt)
  Constant8/1 -> FEM mooring cable/13(Cdn)
  Constant9/1 -> FEM mooring cable/14(depCur)
  Constant3/1 -> FEM mooring cable/15(velCur)
  r0/1 -> mo2/1, FEM mooring cable/1(state)  "[r;r_dot]"
  Constant14/1 -> FEM mooring cable/9(emfact)
  FEM mooring cable/2(Ftop) -> "tau_moor [H_x, H_y, V]"/1, Scope/1, To Workspace2/1
  Constant12/1 -> FEM mooring cable/16(waterDepth)
  Constant15/1 -> FEM mooring cable/2(rBottomEnd)
  Constant17/1 -> FEM mooring cable/10(stiffSeafloor)
  eta/1 -> FEM mooring cable/3(rTopEnd)

== system CSAD_PIDcontroller_ny/Virtual CS Inocean Cat I Drillship 6 DOF/FEM mooring/Mooring Line 3 ==
  eta : Inport
  Constant : Constant  Value=d
  Constant1 : Constant  Value=E
  Constant12 : Constant  Value=waterDepth(3)
  Constant14 : Constant  Value=emfact
  Constant15 : Constant  Value=rBottomEnd(:,3)
  Constant17 : Constant  Value=stiffSeafloor
  Constant2 : Constant  Value=L
  Constant3 : Constant  Value=velCur
  Constant4 : Constant  Value=rhoCab
  Constant5 : Constant  Value=rhoWat
  Constant6 : Constant  Value=Cmn
  Constant7 : Constant  Value=Cdt
  Constant8 : Constant  Value=Cdn
  Constant9 : Constant  Value=depCur
  FEM mooring cable : MATLAB Function  TreatAsAtomicUnit=on
  Scope : Scope
  To Workspace2 : ToWorkspace  VariableName=FtopPlot2  SaveFormat=Timeseries  SampleTime=-1
  mo3 : ToWorkspace  VariableName=mooring_cabel3  SaveFormat=Timeseries  SampleTime=-1
  r0 : Integrator  InitialCondition=[r0(:,3);r_dot0(:,3)]
  "tau_moor [H_x, H_y, V]" : Outport
  wires:
  FEM mooring cable/1(state_dot) -> r0/1  "[r_dot;r_ddot]"
  Constant/1 -> FEM mooring cable/5(d)
  Constant1/1 -> FEM mooring cable/4(E)
  Constant2/1 -> FEM mooring cable/6(L)
  Constant4/1 -> FEM mooring cable/7(rhoCab)
  Constant5/1 -> FEM mooring cable/8(rhoWat)
  Constant6/1 -> FEM mooring cable/11(Cmn)
  Constant7/1 -> FEM mooring cable/12(Cdt)
  Constant8/1 -> FEM mooring cable/13(Cdn)
  Constant9/1 -> FEM mooring cable/14(depCur)
  Constant3/1 -> FEM mooring cable/15(velCur)
  r0/1 -> mo3/1, FEM mooring cable/1(state)  "[r;r_dot]"
  Constant14/1 -> FEM mooring cable/9(emfact)
  FEM mooring cable/2(Ftop) -> "tau_moor [H_x, H_y, V]"/1, Scope/1, To Workspace2/1
  Constant12/1 -> FEM mooring cable/16(waterDepth)
  Constant15/1 -> FEM mooring cable/2(rBottomEnd)
  Constant17/1 -> FEM mooring cable/10(stiffSeafloor)
  eta/1 -> FEM mooring cable/3(rTopEnd)

== system CSAD_PIDcontroller_ny/Virtual CS Inocean Cat I Drillship 6 DOF/FEM mooring/Mooring Line 4 ==
  eta : Inport
  Constant : Constant  Value=d
  Constant1 : Constant  Value=E
  Constant12 : Constant  Value=waterDepth(4)
  Constant14 : Constant  Value=emfact
  Constant15 : Constant  Value=rBottomEnd(:,4)
  Constant17 : Constant  Value=stiffSeafloor
  Constant2 : Constant  Value=L
  Constant3 : Constant  Value=velCur
  Constant4 : Constant  Value=rhoCab
  Constant5 : Constant  Value=rhoWat
  Constant6 : Constant  Value=Cmn
  Constant7 : Constant  Value=Cdt
  Constant8 : Constant  Value=Cdn
  Constant9 : Constant  Value=depCur
  FEM mooring cable : MATLAB Function  TreatAsAtomicUnit=on
  Scope : Scope
  To Workspace2 : ToWorkspace  VariableName=FtopPlot3  SaveFormat=Timeseries  SampleTime=-1
  mo4 : ToWorkspace  VariableName=mooring_cabel4  SaveFormat=Timeseries  SampleTime=-1
  r0 : Integrator  InitialCondition=[r0(:,4);r_dot0(:,4)]
  "tau_moor [H_x, H_y, V]" : Outport
  wires:
  FEM mooring cable/1(state_dot) -> r0/1  "[r_dot;r_ddot]"
  Constant/1 -> FEM mooring cable/5(d)
  Constant1/1 -> FEM mooring cable/4(E)
  Constant2/1 -> FEM mooring cable/6(L)
  Constant4/1 -> FEM mooring cable/7(rhoCab)
  Constant5/1 -> FEM mooring cable/8(rhoWat)
  Constant6/1 -> FEM mooring cable/11(Cmn)
  Constant7/1 -> FEM mooring cable/12(Cdt)
  Constant8/1 -> FEM mooring cable/13(Cdn)
  Constant9/1 -> FEM mooring cable/14(depCur)
  Constant3/1 -> FEM mooring cable/15(velCur)
  r0/1 -> mo4/1, FEM mooring cable/1(state)  "[r;r_dot]"
  Constant14/1 -> FEM mooring cable/9(emfact)
  FEM mooring cable/2(Ftop) -> "tau_moor [H_x, H_y, V]"/1, Scope/1, To Workspace2/1
  Constant12/1 -> FEM mooring cable/16(waterDepth)
  Constant15/1 -> FEM mooring cable/2(rBottomEnd)
  Constant17/1 -> FEM mooring cable/10(stiffSeafloor)
  eta/1 -> FEM mooring cable/3(rTopEnd)

== system CSAD_PIDcontroller_ny/Virtual CS Inocean Cat I Drillship 6 DOF/FEM mooring/Mooring Line 5 ==
  eta : Inport
  Constant : Constant  Value=d
  Constant1 : Constant  Value=E
  Constant12 : Constant  Value=waterDepth(5)
  Constant14 : Constant  Value=emfact
  Constant15 : Constant  Value=rBottomEnd(:,5)
  Constant17 : Constant  Value=stiffSeafloor
  Constant2 : Constant  Value=L
  Constant3 : Constant  Value=velCur
  Constant4 : Constant  Value=rhoCab
  Constant5 : Constant  Value=rhoWat
  Constant6 : Constant  Value=Cmn
  Constant7 : Constant  Value=Cdt
  Constant8 : Constant  Value=Cdn
  Constant9 : Constant  Value=depCur
  FEM mooring cable : MATLAB Function  TreatAsAtomicUnit=on
  Scope : Scope
  To Workspace2 : ToWorkspace  VariableName=FtopPlot4  SaveFormat=Timeseries  SampleTime=-1
  r0 : Integrator  InitialCondition=[r0(:,5);r_dot0(:,5)]
  "tau_moor [H_x, H_y, V]" : Outport
  wires:
  FEM mooring cable/1(state_dot) -> r0/1  "[r_dot;r_ddot]"
  Constant/1 -> FEM mooring cable/5(d)
  Constant1/1 -> FEM mooring cable/4(E)
  Constant2/1 -> FEM mooring cable/6(L)
  Constant4/1 -> FEM mooring cable/7(rhoCab)
  Constant5/1 -> FEM mooring cable/8(rhoWat)
  Constant6/1 -> FEM mooring cable/11(Cmn)
  Constant7/1 -> FEM mooring cable/12(Cdt)
  Constant8/1 -> FEM mooring cable/13(Cdn)
  Constant9/1 -> FEM mooring cable/14(depCur)
  Constant3/1 -> FEM mooring cable/15(velCur)
  r0/1 -> FEM mooring cable/1(state)  "[r;r_dot]"
  Constant14/1 -> FEM mooring cable/9(emfact)
  FEM mooring cable/2(Ftop) -> "tau_moor [H_x, H_y, V]"/1, Scope/1, To Workspace2/1
  Constant12/1 -> FEM mooring cable/16(waterDepth)
  Constant15/1 -> FEM mooring cable/2(rBottomEnd)
  Constant17/1 -> FEM mooring cable/10(stiffSeafloor)
  eta/1 -> FEM mooring cable/3(rTopEnd)

== system CSAD_PIDcontroller_ny/Virtual CS Inocean Cat I Drillship 6 DOF/FEM mooring/Mooring Line 6 ==
  eta : Inport
  Constant : Constant  Value=d
  Constant1 : Constant  Value=E
  Constant12 : Constant  Value=waterDepth(6)
  Constant14 : Constant  Value=emfact
  Constant15 : Constant  Value=rBottomEnd(:,6)
  Constant17 : Constant  Value=stiffSeafloor
  Constant2 : Constant  Value=L
  Constant3 : Constant  Value=velCur
  Constant4 : Constant  Value=rhoCab
  Constant5 : Constant  Value=rhoWat
  Constant6 : Constant  Value=Cmn
  Constant7 : Constant  Value=Cdt
  Constant8 : Constant  Value=Cdn
  Constant9 : Constant  Value=depCur
  FEM mooring cable : MATLAB Function  TreatAsAtomicUnit=on
  Scope : Scope
  To Workspace2 : ToWorkspace  VariableName=FtopPlot5  SaveFormat=Timeseries  SampleTime=-1
  r0 : Integrator  InitialCondition=[r0(:,6);r_dot0(:,6)]
  "tau_moor [H_x, H_y, V]" : Outport
  wires:
  FEM mooring cable/1(state_dot) -> r0/1  "[r_dot;r_ddot]"
  Constant/1 -> FEM mooring cable/5(d)
  Constant1/1 -> FEM mooring cable/4(E)
  Constant2/1 -> FEM mooring cable/6(L)
  Constant4/1 -> FEM mooring cable/7(rhoCab)
  Constant5/1 -> FEM mooring cable/8(rhoWat)
  Constant6/1 -> FEM mooring cable/11(Cmn)
  Constant7/1 -> FEM mooring cable/12(Cdt)
  Constant8/1 -> FEM mooring cable/13(Cdn)
  Constant9/1 -> FEM mooring cable/14(depCur)
  Constant3/1 -> FEM mooring cable/15(velCur)
  r0/1 -> FEM mooring cable/1(state)  "[r;r_dot]"
  Constant14/1 -> FEM mooring cable/9(emfact)
  FEM mooring cable/2(Ftop) -> "tau_moor [H_x, H_y, V]"/1, Scope/1, To Workspace2/1
  Constant12/1 -> FEM mooring cable/16(waterDepth)
  Constant15/1 -> FEM mooring cable/2(rBottomEnd)
  Constant17/1 -> FEM mooring cable/10(stiffSeafloor)
  eta/1 -> FEM mooring cable/3(rTopEnd)

== system CSAD_PIDcontroller_ny/Virtual CS Inocean Cat I Drillship 6 DOF/FEM mooring/Mooring Line 7 ==
  eta : Inport
  Constant : Constant  Value=d
  Constant1 : Constant  Value=E
  Constant12 : Constant  Value=waterDepth(7)
  Constant14 : Constant  Value=emfact
  Constant15 : Constant  Value=rBottomEnd(:,7)
  Constant17 : Constant  Value=stiffSeafloor
  Constant2 : Constant  Value=L
  Constant3 : Constant  Value=velCur
  Constant4 : Constant  Value=rhoCab
  Constant5 : Constant  Value=rhoWat
  Constant6 : Constant  Value=Cmn
  Constant7 : Constant  Value=Cdt
  Constant8 : Constant  Value=Cdn
  Constant9 : Constant  Value=depCur
  FEM mooring cable : MATLAB Function  TreatAsAtomicUnit=on
  Scope : Scope
  To Workspace2 : ToWorkspace  VariableName=FtopPlot6  SaveFormat=Timeseries  SampleTime=-1
  r0 : Integrator  InitialCondition=[r0(:,7);r_dot0(:,7)]
  "tau_moor [H_x, H_y, V]" : Outport
  wires:
  FEM mooring cable/1(state_dot) -> r0/1  "[r_dot;r_ddot]"
  Constant/1 -> FEM mooring cable/5(d)
  Constant1/1 -> FEM mooring cable/4(E)
  Constant2/1 -> FEM mooring cable/6(L)
  Constant4/1 -> FEM mooring cable/7(rhoCab)
  Constant5/1 -> FEM mooring cable/8(rhoWat)
  Constant6/1 -> FEM mooring cable/11(Cmn)
  Constant7/1 -> FEM mooring cable/12(Cdt)
  Constant8/1 -> FEM mooring cable/13(Cdn)
  Constant9/1 -> FEM mooring cable/14(depCur)
  Constant3/1 -> FEM mooring cable/15(velCur)
  r0/1 -> FEM mooring cable/1(state)  "[r;r_dot]"
  Constant14/1 -> FEM mooring cable/9(emfact)
  FEM mooring cable/2(Ftop) -> "tau_moor [H_x, H_y, V]"/1, Scope/1, To Workspace2/1
  Constant12/1 -> FEM mooring cable/16(waterDepth)
  Constant15/1 -> FEM mooring cable/2(rBottomEnd)
  Constant17/1 -> FEM mooring cable/10(stiffSeafloor)
  eta/1 -> FEM mooring cable/3(rTopEnd)
